simulink model "bpsk_cos"  (Simulink 6.4)
settings: Solver=FixedStepDiscrete  StartTime=0.0  StopTime=12  RelTol=1e-3
undefined symbols (not defined in the file or in its folder): Fs, get
libraries: commsink2 x3, commdigbbndpm3 x2, commfilt2 x2, commchan3 x1, dspsrcs4 x1, dspsigops x1, commrandsrc2 x1, dspsnks4 x1
settings Model: Creator=ALEX  LastModifiedBy=student
settings OptimizationCC: InitFltsAndDblsToZero=off
settings DebuggingCC: SignalResolutionControl=UseLocalSettings  MultiTaskDSMMsg=error  MultiTaskCondExecSysMsg=error
settings GRTTargetCC: TargetFcnLib=ansi_tfl_table_tmw.mat

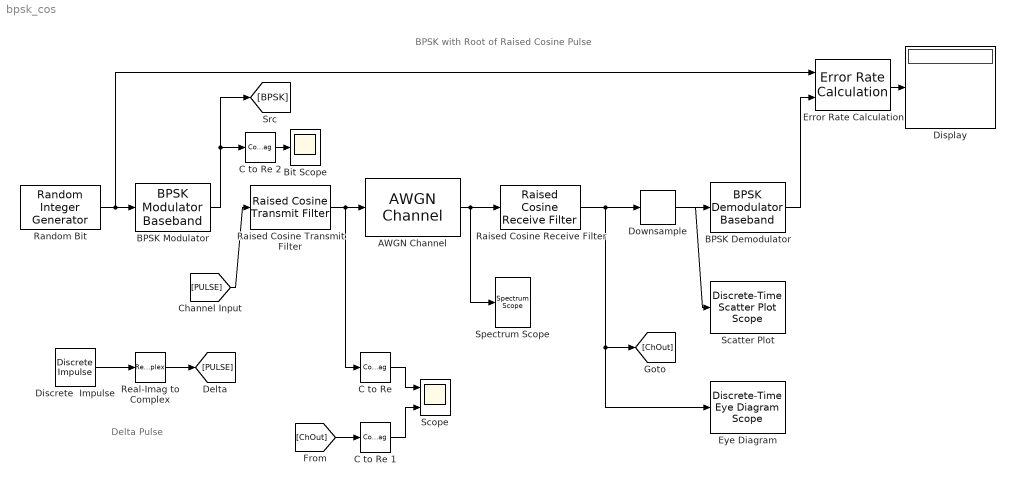
== system bpsk_cos ==
  note: BPSK with Root of Raised Cosine Pulse
  note: Delta Pulse
  AWGN Channel : commchan3/AWGN Channel  SystemSampleTime=-1  seed=67  noiseMode="Signal to noise ratio  (Es/No)"  EbNodB=3  EsNodB=100  SNRdB=10  bitsPerSym=1  Ps=1/16  Tsym=1  variance=0
  BPSK Demodulator : commdigbbndpm3/BPSK Demodulator Baseband  SystemSampleTime=-1  Ph=0  outDtype=boolean
  BPSK Modulator : commdigbbndpm3/BPSK Modulator Baseband  SystemSampleTime=-1  Ph=0  outDtype=double  outWordLen=16  outUDDataType=sfix(16)  outFracLenMode=Best precision  outFracLen=15
  Bit Scope : Scope
      settings: TimeRange=16  YMin=-1.2  YMax=1.2  SampleTime=1/64
  C to Re : ComplexToRealImag  Output=Real
  C to Re 1 : ComplexToRealImag  Output=Real
  C to Re 2 : ComplexToRealImag  Output=Real
  Discrete  Impulse : dspsrcs4/Discrete  Impulse  Delay=0  SampleTime=1  FrameSample=1  dataType=double  isSigned=on  wordLen=16  udDataType=sfix(16)  fracBitsMode=Best precision  numFracBits=15
  Display : Display
  Downsample : dspsigops/Downsample  N=16  phase=0  ic=0  smode=Allow multirate  fmode=Maintain input frame size
  Error Rate Calculation : commsink2/Error Rate Calculation  N=10  st_delay=0  cp_mode=Entire frame  subframe=[]  PMode=Port  WsName=ErrorVec  RsMode2=off  stop=off  numErr=100  maxBits=100000
  Eye Diagram : commsink2/Discrete-Time Eye Diagram Scope  Tag=EyeDiagram  SystemSampleTime=-1  sampPerSymb=16  offsetEye=0  symbPerTrace=2  numTraces=40  numNewFrames=10  LineStyles=-  LineColors=b  dupPoints=on  fading=on  render=on  AxisGrid=on  yMin=-3  yMax=3  inphaseLabel=In-phase Amplitude  quadratureLabel=Quadrature Amplitude  openScopeAtSimStart=off  dispDiagram=In-phase Only  FrameNumber=off  FigPos=[360 435 560 487]  figTitle=Eye Diagram  block_type_=eye  numLinesMax=8
  Raised Cosine Receive Filter : commfilt2/Raised Cosine Receive Filter  DialogController=dspDDGCreate  DialogControllerArgs=DataTag0  SystemSampleTime=-1  filtType=Square root  N=16  D=4  R=0.5  sampMode=Sample-based  rateMode=None  downFactor=16  downOffset=0  checkGain=Normalized  filterGain=1  checkCoeff=off  variableName=rcRxFilt  launchFVT=off
  Raised Cosine Transmit Filter : commfilt2/Raised Cosine Transmit Filter  DialogController=dspDDGCreate  DialogControllerArgs=DataTag1  SystemSampleTime=-1  filtType=Square root  D=4  R=0.5  sampMode=Sample-based  N=16  checkGain=Normalized  filterGain=1  checkCoeff=on  variableName=rcTxFilt  launchFVT=off
  Random Bit : commrandsrc2/Random Integer Generator  SystemSampleTime=-1  mul=2  seed=67  Ts=1  frameBased=off  sampPerFrame=8  orient=off  outDataType=boolean
  Real-Imag to Complex : RealImagToComplex  Input=Real
  Scatter Plot : commsink2/Discrete-Time Scatter Plot Scope  Tag=ScatterPlot  SystemSampleTime=-1  sampPerSymb=1  offsetEye=0  numTraces=40  numNewFrames=10  LineMarkers=.  LineColors=b  fading=on  render=on  AxisGrid=on  xMin=-2  xMax=2  yMin=-2  yMax=2  inphaseLabel=In-phase Amplitude  quadratureLabel=Quadrature Amplitude  openScopeAtSimStart=off  FrameNumber=off  FigPos=[360 435 560 487]  figTitle=Scatter Plot  numLinesMax=8  block_type_=scatter
  Scope : Scope  NumInputPorts=2
      settings: TimeRange=16  YMin=-0.4~-1.5  YMax=0.4~1.5  SampleTime=1/64
  Spectrum Scope : dspsnks4/Spectrum Scope  DialogController=dspdialog.SpectrumScope  DialogControllerArgs=DataTag2  SystemSampleTime=-1  ScopeProperties=on  Domain=Frequency  HorizSpan=1  UseBuffer=on  BufferSize=2048  Overlap=0  inpFftLenInherit=off  FFTlength=1024  numAvg=50  DisplayProperties=off  AxisGrid=on  Memory=off  FrameNumber=on  AxisLegend=off  AxisZoom=off  OpenScopeAtSimStart=off  OpenScopeImmediately=off  FigPos=get(0,'defaultfigureposition')  AxisProperties=off  XUnits=Hertz  XRange=[-Fs/2...Fs/2]  InheritXIncr=on  XIncr=1.0  XLabel=Samples  YUnits=dB  YLabel=Magnitude-squared, dB  LineProperties=off  LineMarkers=None  wintypeSpecScope=Hamming  RsSpecScope=50  betaSpecScope=5  winsampSpecScope=Periodic
      settings: YMin=-72.0061  YMax=2.2739
  wires:
  Error Rate Calculation/1 -> Display/1
  Random Bit/1 -> BPSK Modulator/1, Error Rate Calculation/1
  Raised Cosine Transmit Filter/1 -> AWGN Channel/1, C to Re/1
  AWGN Channel/1 -> Spectrum Scope/1, Raised Cosine Receive Filter/1
  Raised Cosine Receive Filter/1 -> Downsample/1, [ChOut], Eye Diagram/1
  BPSK Demodulator/1 -> Error Rate Calculation/2
  Downsample/1 -> BPSK Demodulator/1, Scatter Plot/1
  Discrete  Impulse/1 -> Real-Imag to Complex/1
  C to Re/1 -> Scope/1
  C to Re 1/1 -> Scope/2
  [ChOut] -> C to Re 1/1
  C to Re 2/1 -> Bit Scope/1
  BPSK Modulator/1 -> [BPSK], C to Re 2/1
  Real-Imag to Complex/1 -> [PULSE]
  [PULSE] -> Raised Cosine Transmit Filter/1
